simulink model "PRACTICA_03_P1_00"  (R2022a)
settings: Solver=VariableStepAuto  StartTime=0.0  StopTime=10.0  RelTol=1e-3
undefined symbols (not defined in the file or in its folder): xc7z010iclg225
libraries: hdlBasic x889, vmcUtilities x1
(part 2 of 4)

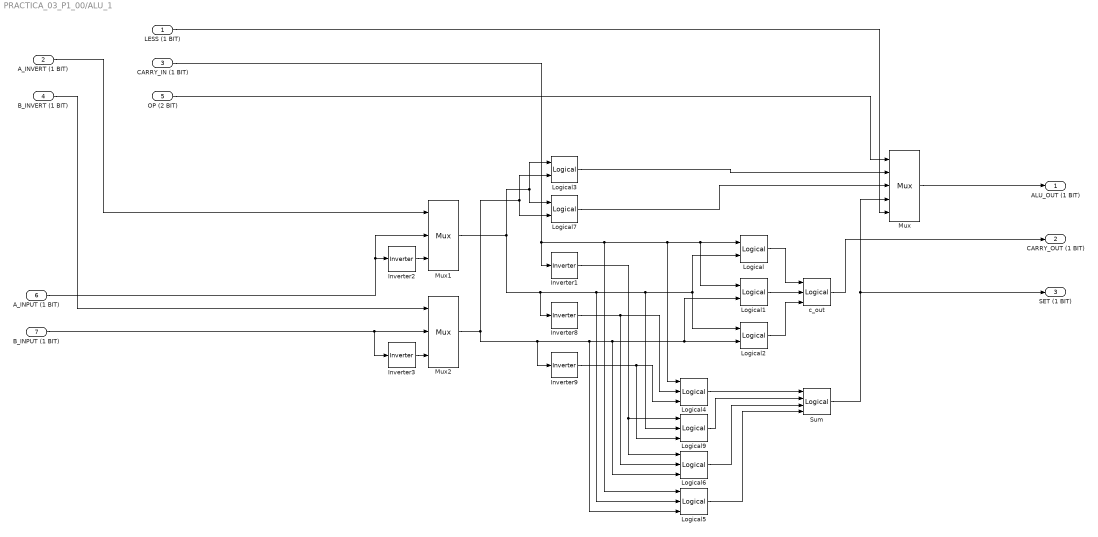
== system PRACTICA_03_P1_00/ALU_1 ==
  LESS (1 BIT) : Inport
  A_INVERT (1 BIT) : Inport  Port=2
  CARRY_IN (1 BIT) : Inport  Port=3
  B_INVERT (1 BIT) : Inport  Port=4
  OP (2 BIT) : Inport  Port=5
  A_INPUT (1 BIT) : Inport  Port=6
  B_INPUT (1 BIT) : Inport  Port=7
  Inverter{1..3,8..9} (5 alike) : hdlBasic/Inverter  en=off  latency=0  XmcBlockStatus=1  maskContainerNames=group2  block_type=inv  block_config=sysgen:Inverter_config
  Logical{,1..3} (4 alike) : hdlBasic/Logical  logical_function=AND  inputs=2  en=off  latency=0  precision=Full  arith_type=Unsigned  n_bits=16  bin_pt=0  align_bp=on  overflow=[]  quantization=[]  XmcBlockStatus=1  maskContainerNames=tabcontainer1  block_type=logical  block_config=sysgen:Logical_config
  Logical{4..6,9} (4 alike) : hdlBasic/Logical  logical_function=AND  inputs=3  en=off  latency=0  precision=Full  arith_type=Unsigned  n_bits=16  bin_pt=0  align_bp=on  overflow=[]  quantization=[]  XmcBlockStatus=1  maskContainerNames=tabcontainer1  block_type=logical  block_config=sysgen:Logical_config
  Logical7 : hdlBasic/Logical  logical_function=OR  inputs=2  en=off  latency=0  precision=Full  arith_type=Unsigned  n_bits=16  bin_pt=0  align_bp=on  overflow=[]  quantization=[]  XmcBlockStatus=1  maskContainerNames=tabcontainer1  block_type=logical  block_config=sysgen:Logical_config
  Mux : hdlBasic/Mux  inputs=4  en=off  latency=0  precision=Full  arith_type=Unsigned  n_bits=16  bin_pt=14  quantization=Truncate  overflow=Wrap  XmcBlockStatus=1  maskContainerNames=tabcontainer1  block_type=mux  block_config=sysgen:Mux_config
  Mux1 : hdlBasic/Mux  inputs=2  en=off  latency=0  precision=Full  arith_type=Unsigned  n_bits=16  bin_pt=14  quantization=Truncate  overflow=Wrap  XmcBlockStatus=1  maskContainerNames=tabcontainer1  block_type=mux  block_config=sysgen:Mux_config
  Mux2 : hdlBasic/Mux  inputs=2  en=off  latency=0  precision=Full  arith_type=Unsigned  n_bits=16  bin_pt=14  quantization=Truncate  overflow=Wrap  XmcBlockStatus=1  maskContainerNames=tabcontainer1  block_type=mux  block_config=sysgen:Mux_config
  Sum : hdlBasic/Logical  logical_function=OR  inputs=4  en=off  latency=0  precision=Full  arith_type=Unsigned  n_bits=16  bin_pt=0  align_bp=on  overflow=[]  quantization=[]  XmcBlockStatus=1  maskContainerNames=tabcontainer1  block_type=logical  block_config=sysgen:Logical_config
  c_out : hdlBasic/Logical  logical_function=OR  inputs=3  en=off  latency=0  precision=Full  arith_type=Unsigned  n_bits=16  bin_pt=0  align_bp=on  overflow=[]  quantization=[]  XmcBlockStatus=1  maskContainerNames=tabcontainer1  block_type=logical  block_config=sysgen:Logical_config
  ALU_OUT (1 BIT) : Outport
  CARRY_OUT (1 BIT) : Outport  Port=2
  SET (1 BIT) : Outport  Port=3
  wires:
  Mux1/1 -> Logical3/1, Logical7/1, Inverter8/1, Logical5/2, Logical/2, Logical2/1, Logical9/2
  Logical1/1 -> c_out/2
  Inverter8/1 -> Logical6/2, Logical4/2
  A_INPUT (1 BIT)/1 -> Mux1/2, Inverter2/1
  CARRY_IN (1 BIT)/1 -> Inverter1/1, Logical5/1, Logical4/1, Logical1/1, Logical/1
  Mux2/1 -> Logical5/3, Logical6/3, Logical1/2, Logical2/2, Inverter9/1, Logical3/2, Logical7/2
  Inverter2/1 -> Mux1/3
  Inverter1/1 -> Logical6/1, Logical9/1
  Logical6/1 -> Sum/3
  B_INPUT (1 BIT)/1 -> Inverter3/1, Mux2/2
  Logical9/1 -> Sum/2
  Sum/1 -> SET (1 BIT)/1, Mux/4
  Logical4/1 -> Sum/1
  Inverter3/1 -> Mux2/3
  Logical7/1 -> Mux/3
  Logical/1 -> c_out/1
  Logical5/1 -> Sum/4
  Logical3/1 -> Mux/2
  Inverter9/1 -> Logical9/3, Logical4/3
  Mux/1 -> ALU_OUT (1 BIT)/1
  Logical2/1 -> c_out/3
  OP (2 BIT)/1 -> Mux/1
  A_INVERT (1 BIT)/1 -> Mux1/1
  B_INVERT (1 BIT)/1 -> Mux2/1
  c_out/1 -> CARRY_OUT (1 BIT)/1
  LESS (1 BIT)/1 -> Mux/5

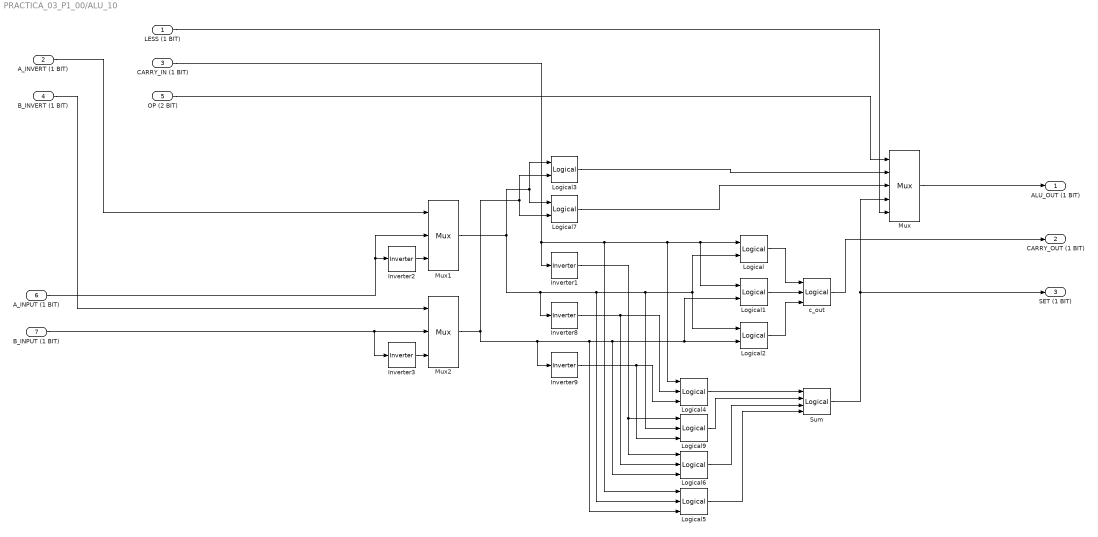
== system PRACTICA_03_P1_00/ALU_10 ==
  LESS (1 BIT) : Inport
  A_INVERT (1 BIT) : Inport  Port=2
  CARRY_IN (1 BIT) : Inport  Port=3
  B_INVERT (1 BIT) : Inport  Port=4
  OP (2 BIT) : Inport  Port=5
  A_INPUT (1 BIT) : Inport  Port=6
  B_INPUT (1 BIT) : Inport  Port=7
  Inverter{1..3,8..9} (5 alike) : hdlBasic/Inverter  en=off  latency=0  XmcBlockStatus=1  maskContainerNames=group2  block_type=inv  block_config=sysgen:Inverter_config
  Logical{,1..3} (4 alike) : hdlBasic/Logical  logical_function=AND  inputs=2  en=off  latency=0  precision=Full  arith_type=Unsigned  n_bits=16  bin_pt=0  align_bp=on  overflow=[]  quantization=[]  XmcBlockStatus=1  maskContainerNames=tabcontainer1  block_type=logical  block_config=sysgen:Logical_config
  Logical{4..6,9} (4 alike) : hdlBasic/Logical  logical_function=AND  inputs=3  en=off  latency=0  precision=Full  arith_type=Unsigned  n_bits=16  bin_pt=0  align_bp=on  overflow=[]  quantization=[]  XmcBlockStatus=1  maskContainerNames=tabcontainer1  block_type=logical  block_config=sysgen:Logical_config
  Logical7 : hdlBasic/Logical  logical_function=OR  inputs=2  en=off  latency=0  precision=Full  arith_type=Unsigned  n_bits=16  bin_pt=0  align_bp=on  overflow=[]  quantization=[]  XmcBlockStatus=1  maskContainerNames=tabcontainer1  block_type=logical  block_config=sysgen:Logical_config
  Mux : hdlBasic/Mux  inputs=4  en=off  latency=0  precision=Full  arith_type=Unsigned  n_bits=16  bin_pt=14  quantization=Truncate  overflow=Wrap  XmcBlockStatus=1  maskContainerNames=tabcontainer1  block_type=mux  block_config=sysgen:Mux_config
  Mux1 : hdlBasic/Mux  inputs=2  en=off  latency=0  precision=Full  arith_type=Unsigned  n_bits=16  bin_pt=14  quantization=Truncate  overflow=Wrap  XmcBlockStatus=1  maskContainerNames=tabcontainer1  block_type=mux  block_config=sysgen:Mux_config
  Mux2 : hdlBasic/Mux  inputs=2  en=off  latency=0  precision=Full  arith_type=Unsigned  n_bits=16  bin_pt=14  quantization=Truncate  overflow=Wrap  XmcBlockStatus=1  maskContainerNames=tabcontainer1  block_type=mux  block_config=sysgen:Mux_config
  Sum : hdlBasic/Logical  logical_function=OR  inputs=4  en=off  latency=0  precision=Full  arith_type=Unsigned  n_bits=16  bin_pt=0  align_bp=on  overflow=[]  quantization=[]  XmcBlockStatus=1  maskContainerNames=tabcontainer1  block_type=logical  block_config=sysgen:Logical_config
  c_out : hdlBasic/Logical  logical_function=OR  inputs=3  en=off  latency=0  precision=Full  arith_type=Unsigned  n_bits=16  bin_pt=0  align_bp=on  overflow=[]  quantization=[]  XmcBlockStatus=1  maskContainerNames=tabcontainer1  block_type=logical  block_config=sysgen:Logical_config
  ALU_OUT (1 BIT) : Outport
  CARRY_OUT (1 BIT) : Outport  Port=2
  SET (1 BIT) : Outport  Port=3
  wires:
  Mux1/1 -> Logical3/1, Logical7/1, Inverter8/1, Logical5/2, Logical/2, Logical2/1, Logical9/2
  Logical1/1 -> c_out/2
  Inverter8/1 -> Logical6/2, Logical4/2
  A_INPUT (1 BIT)/1 -> Mux1/2, Inverter2/1
  CARRY_IN (1 BIT)/1 -> Inverter1/1, Logical5/1, Logical4/1, Logical1/1, Logical/1
  Mux2/1 -> Logical5/3, Logical6/3, Logical1/2, Logical2/2, Inverter9/1, Logical3/2, Logical7/2
  Inverter2/1 -> Mux1/3
  Inverter1/1 -> Logical6/1, Logical9/1
  Logical6/1 -> Sum/3
  B_INPUT (1 BIT)/1 -> Inverter3/1, Mux2/2
  Logical9/1 -> Sum/2
  Sum/1 -> SET (1 BIT)/1, Mux/4
  Logical4/1 -> Sum/1
  Inverter3/1 -> Mux2/3
  Logical7/1 -> Mux/3
  Logical/1 -> c_out/1
  Logical5/1 -> Sum/4
  Logical3/1 -> Mux/2
  Inverter9/1 -> Logical9/3, Logical4/3
  Mux/1 -> ALU_OUT (1 BIT)/1
  Logical2/1 -> c_out/3
  OP (2 BIT)/1 -> Mux/1
  A_INVERT (1 BIT)/1 -> Mux1/1
  B_INVERT (1 BIT)/1 -> Mux2/1
  c_out/1 -> CARRY_OUT (1 BIT)/1
  LESS (1 BIT)/1 -> Mux/5

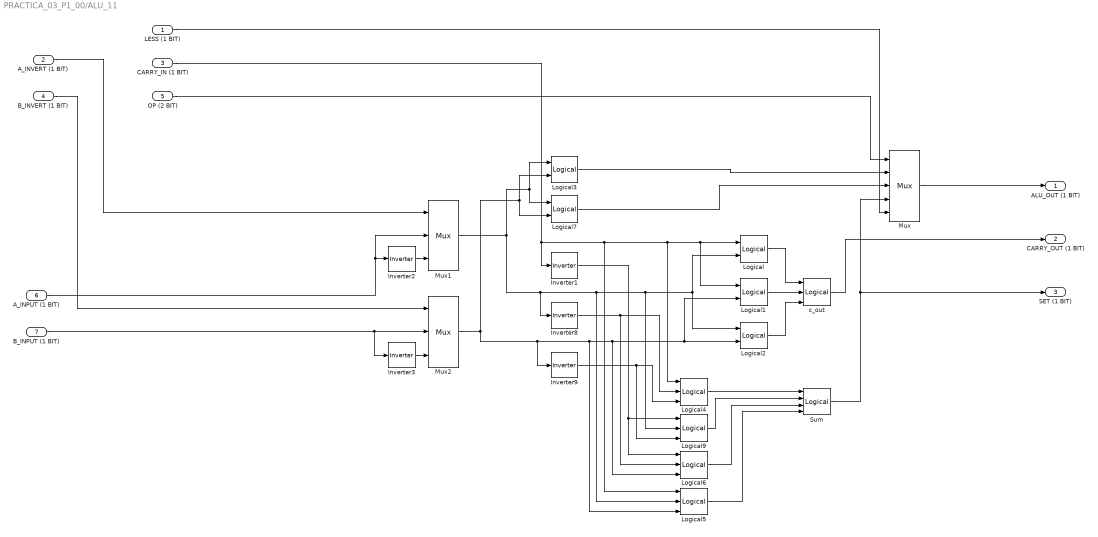
== system PRACTICA_03_P1_00/ALU_11 ==
  LESS (1 BIT) : Inport
  A_INVERT (1 BIT) : Inport  Port=2
  CARRY_IN (1 BIT) : Inport  Port=3
  B_INVERT (1 BIT) : Inport  Port=4
  OP (2 BIT) : Inport  Port=5
  A_INPUT (1 BIT) : Inport  Port=6
  B_INPUT (1 BIT) : Inport  Port=7
  Inverter{1..3,8..9} (5 alike) : hdlBasic/Inverter  en=off  latency=0  XmcBlockStatus=1  maskContainerNames=group2  block_type=inv  block_config=sysgen:Inverter_config
  Logical{,1..3} (4 alike) : hdlBasic/Logical  logical_function=AND  inputs=2  en=off  latency=0  precision=Full  arith_type=Unsigned  n_bits=16  bin_pt=0  align_bp=on  overflow=[]  quantization=[]  XmcBlockStatus=1  maskContainerNames=tabcontainer1  block_type=logical  block_config=sysgen:Logical_config
  Logical{4..6,9} (4 alike) : hdlBasic/Logical  logical_function=AND  inputs=3  en=off  latency=0  precision=Full  arith_type=Unsigned  n_bits=16  bin_pt=0  align_bp=on  overflow=[]  quantization=[]  XmcBlockStatus=1  maskContainerNames=tabcontainer1  block_type=logical  block_config=sysgen:Logical_config
  Logical7 : hdlBasic/Logical  logical_function=OR  inputs=2  en=off  latency=0  precision=Full  arith_type=Unsigned  n_bits=16  bin_pt=0  align_bp=on  overflow=[]  quantization=[]  XmcBlockStatus=1  maskContainerNames=tabcontainer1  block_type=logical  block_config=sysgen:Logical_config
  Mux : hdlBasic/Mux  inputs=4  en=off  latency=0  precision=Full  arith_type=Unsigned  n_bits=16  bin_pt=14  quantization=Truncate  overflow=Wrap  XmcBlockStatus=1  maskContainerNames=tabcontainer1  block_type=mux  block_config=sysgen:Mux_config
  Mux1 : hdlBasic/Mux  inputs=2  en=off  latency=0  precision=Full  arith_type=Unsigned  n_bits=16  bin_pt=14  quantization=Truncate  overflow=Wrap  XmcBlockStatus=1  maskContainerNames=tabcontainer1  block_type=mux  block_config=sysgen:Mux_config
  Mux2 : hdlBasic/Mux  inputs=2  en=off  latency=0  precision=Full  arith_type=Unsigned  n_bits=16  bin_pt=14  quantization=Truncate  overflow=Wrap  XmcBlockStatus=1  maskContainerNames=tabcontainer1  block_type=mux  block_config=sysgen:Mux_config
  Sum : hdlBasic/Logical  logical_function=OR  inputs=4  en=off  latency=0  precision=Full  arith_type=Unsigned  n_bits=16  bin_pt=0  align_bp=on  overflow=[]  quantization=[]  XmcBlockStatus=1  maskContainerNames=tabcontainer1  block_type=logical  block_config=sysgen:Logical_config
  c_out : hdlBasic/Logical  logical_function=OR  inputs=3  en=off  latency=0  precision=Full  arith_type=Unsigned  n_bits=16  bin_pt=0  align_bp=on  overflow=[]  quantization=[]  XmcBlockStatus=1  maskContainerNames=tabcontainer1  block_type=logical  block_config=sysgen:Logical_config
  ALU_OUT (1 BIT) : Outport
  CARRY_OUT (1 BIT) : Outport  Port=2
  SET (1 BIT) : Outport  Port=3
  wires:
  Mux1/1 -> Logical3/1, Logical7/1, Inverter8/1, Logical5/2, Logical/2, Logical2/1, Logical9/2
  Logical1/1 -> c_out/2
  Inverter8/1 -> Logical6/2, Logical4/2
  A_INPUT (1 BIT)/1 -> Mux1/2, Inverter2/1
  CARRY_IN (1 BIT)/1 -> Inverter1/1, Logical5/1, Logical4/1, Logical1/1, Logical/1
  Mux2/1 -> Logical5/3, Logical6/3, Logical1/2, Logical2/2, Inverter9/1, Logical3/2, Logical7/2
  Inverter2/1 -> Mux1/3
  Inverter1/1 -> Logical6/1, Logical9/1
  Logical6/1 -> Sum/3
  B_INPUT (1 BIT)/1 -> Inverter3/1, Mux2/2
  Logical9/1 -> Sum/2
  Sum/1 -> SET (1 BIT)/1, Mux/4
  Logical4/1 -> Sum/1
  Inverter3/1 -> Mux2/3
  Logical7/1 -> Mux/3
  Logical/1 -> c_out/1
  Logical5/1 -> Sum/4
  Logical3/1 -> Mux/2
  Inverter9/1 -> Logical9/3, Logical4/3
  Mux/1 -> ALU_OUT (1 BIT)/1
  Logical2/1 -> c_out/3
  OP (2 BIT)/1 -> Mux/1
  A_INVERT (1 BIT)/1 -> Mux1/1
  B_INVERT (1 BIT)/1 -> Mux2/1
  c_out/1 -> CARRY_OUT (1 BIT)/1
  LESS (1 BIT)/1 -> Mux/5

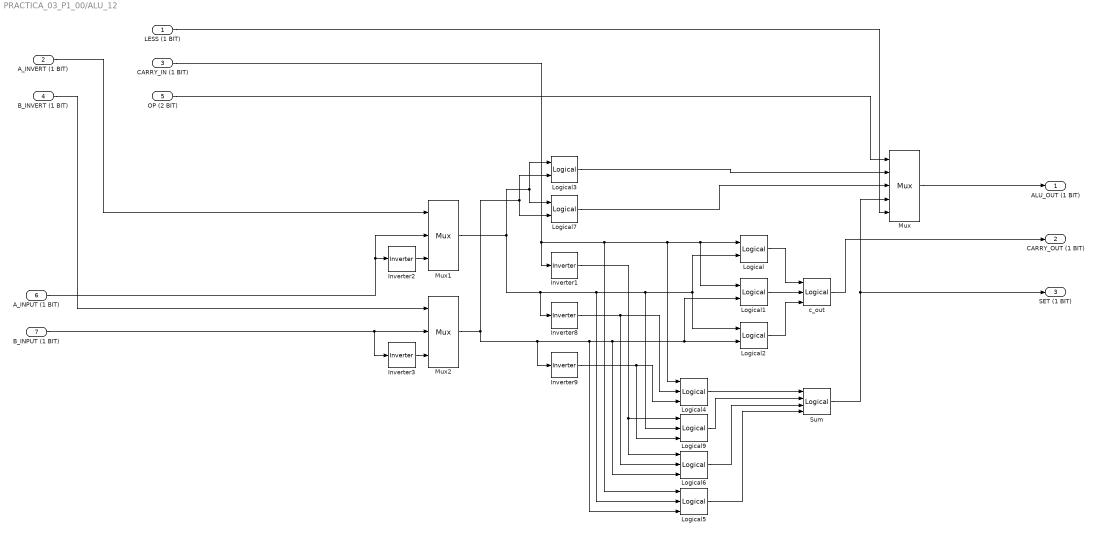
== system PRACTICA_03_P1_00/ALU_12 ==
  LESS (1 BIT) : Inport
  A_INVERT (1 BIT) : Inport  Port=2
  CARRY_IN (1 BIT) : Inport  Port=3
  B_INVERT (1 BIT) : Inport  Port=4
  OP (2 BIT) : Inport  Port=5
  A_INPUT (1 BIT) : Inport  Port=6
  B_INPUT (1 BIT) : Inport  Port=7
  Inverter{1..3,8..9} (5 alike) : hdlBasic/Inverter  en=off  latency=0  XmcBlockStatus=1  maskContainerNames=group2  block_type=inv  block_config=sysgen:Inverter_config
  Logical{,1..3} (4 alike) : hdlBasic/Logical  logical_function=AND  inputs=2  en=off  latency=0  precision=Full  arith_type=Unsigned  n_bits=16  bin_pt=0  align_bp=on  overflow=[]  quantization=[]  XmcBlockStatus=1  maskContainerNames=tabcontainer1  block_type=logical  block_config=sysgen:Logical_config
  Logical{4..6,9} (4 alike) : hdlBasic/Logical  logical_function=AND  inputs=3  en=off  latency=0  precision=Full  arith_type=Unsigned  n_bits=16  bin_pt=0  align_bp=on  overflow=[]  quantization=[]  XmcBlockStatus=1  maskContainerNames=tabcontainer1  block_type=logical  block_config=sysgen:Logical_config
  Logical7 : hdlBasic/Logical  logical_function=OR  inputs=2  en=off  latency=0  precision=Full  arith_type=Unsigned  n_bits=16  bin_pt=0  align_bp=on  overflow=[]  quantization=[]  XmcBlockStatus=1  maskContainerNames=tabcontainer1  block_type=logical  block_config=sysgen:Logical_config
  Mux : hdlBasic/Mux  inputs=4  en=off  latency=0  precision=Full  arith_type=Unsigned  n_bits=16  bin_pt=14  quantization=Truncate  overflow=Wrap  XmcBlockStatus=1  maskContainerNames=tabcontainer1  block_type=mux  block_config=sysgen:Mux_config
  Mux1 : hdlBasic/Mux  inputs=2  en=off  latency=0  precision=Full  arith_type=Unsigned  n_bits=16  bin_pt=14  quantization=Truncate  overflow=Wrap  XmcBlockStatus=1  maskContainerNames=tabcontainer1  block_type=mux  block_config=sysgen:Mux_config
  Mux2 : hdlBasic/Mux  inputs=2  en=off  latency=0  precision=Full  arith_type=Unsigned  n_bits=16  bin_pt=14  quantization=Truncate  overflow=Wrap  XmcBlockStatus=1  maskContainerNames=tabcontainer1  block_type=mux  block_config=sysgen:Mux_config
  Sum : hdlBasic/Logical  logical_function=OR  inputs=4  en=off  latency=0  precision=Full  arith_type=Unsigned  n_bits=16  bin_pt=0  align_bp=on  overflow=[]  quantization=[]  XmcBlockStatus=1  maskContainerNames=tabcontainer1  block_type=logical  block_config=sysgen:Logical_config
  c_out : hdlBasic/Logical  logical_function=OR  inputs=3  en=off  latency=0  precision=Full  arith_type=Unsigned  n_bits=16  bin_pt=0  align_bp=on  overflow=[]  quantization=[]  XmcBlockStatus=1  maskContainerNames=tabcontainer1  block_type=logical  block_config=sysgen:Logical_config
  ALU_OUT (1 BIT) : Outport
  CARRY_OUT (1 BIT) : Outport  Port=2
  SET (1 BIT) : Outport  Port=3
  wires:
  Mux1/1 -> Logical3/1, Logical7/1, Inverter8/1, Logical5/2, Logical/2, Logical2/1, Logical9/2
  Logical1/1 -> c_out/2
  Inverter8/1 -> Logical6/2, Logical4/2
  A_INPUT (1 BIT)/1 -> Mux1/2, Inverter2/1
  CARRY_IN (1 BIT)/1 -> Inverter1/1, Logical5/1, Logical4/1, Logical1/1, Logical/1
  Mux2/1 -> Logical5/3, Logical6/3, Logical1/2, Logical2/2, Inverter9/1, Logical3/2, Logical7/2
  Inverter2/1 -> Mux1/3
  Inverter1/1 -> Logical6/1, Logical9/1
  Logical6/1 -> Sum/3
  B_INPUT (1 BIT)/1 -> Inverter3/1, Mux2/2
  Logical9/1 -> Sum/2
  Sum/1 -> SET (1 BIT)/1, Mux/4
  Logical4/1 -> Sum/1
  Inverter3/1 -> Mux2/3
  Logical7/1 -> Mux/3
  Logical/1 -> c_out/1
  Logical5/1 -> Sum/4
  Logical3/1 -> Mux/2
  Inverter9/1 -> Logical9/3, Logical4/3
  Mux/1 -> ALU_OUT (1 BIT)/1
  Logical2/1 -> c_out/3
  OP (2 BIT)/1 -> Mux/1
  A_INVERT (1 BIT)/1 -> Mux1/1
  B_INVERT (1 BIT)/1 -> Mux2/1
  c_out/1 -> CARRY_OUT (1 BIT)/1
  LESS (1 BIT)/1 -> Mux/5

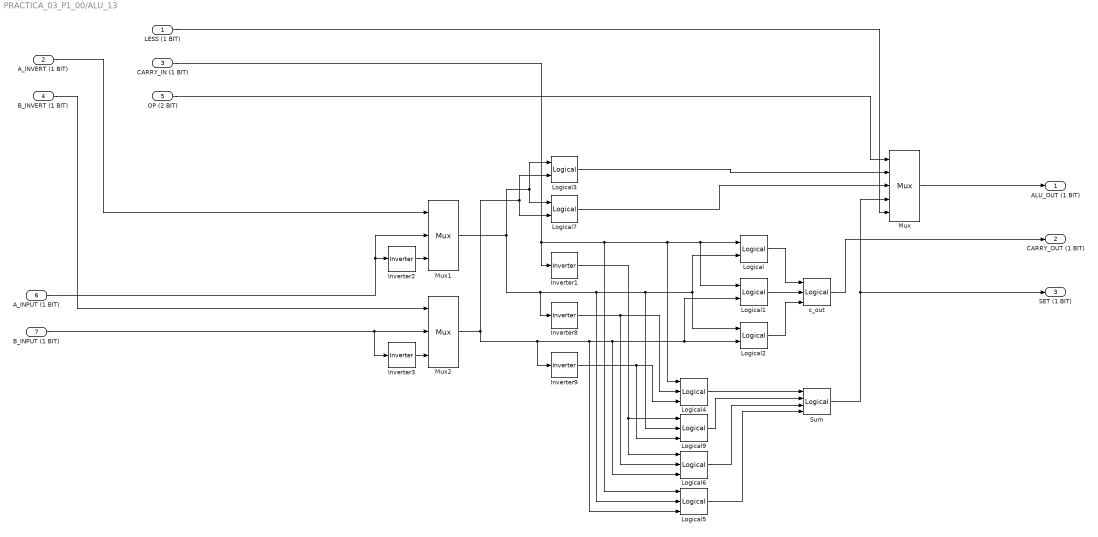
== system PRACTICA_03_P1_00/ALU_13 ==
  LESS (1 BIT) : Inport
  A_INVERT (1 BIT) : Inport  Port=2
  CARRY_IN (1 BIT) : Inport  Port=3
  B_INVERT (1 BIT) : Inport  Port=4
  OP (2 BIT) : Inport  Port=5
  A_INPUT (1 BIT) : Inport  Port=6
  B_INPUT (1 BIT) : Inport  Port=7
  Inverter{1..3,8..9} (5 alike) : hdlBasic/Inverter  en=off  latency=0  XmcBlockStatus=1  maskContainerNames=group2  block_type=inv  block_config=sysgen:Inverter_config
  Logical{,1..3} (4 alike) : hdlBasic/Logical  logical_function=AND  inputs=2  en=off  latency=0  precision=Full  arith_type=Unsigned  n_bits=16  bin_pt=0  align_bp=on  overflow=[]  quantization=[]  XmcBlockStatus=1  maskContainerNames=tabcontainer1  block_type=logical  block_config=sysgen:Logical_config
  Logical{4..6,9} (4 alike) : hdlBasic/Logical  logical_function=AND  inputs=3  en=off  latency=0  precision=Full  arith_type=Unsigned  n_bits=16  bin_pt=0  align_bp=on  overflow=[]  quantization=[]  XmcBlockStatus=1  maskContainerNames=tabcontainer1  block_type=logical  block_config=sysgen:Logical_config
  Logical7 : hdlBasic/Logical  logical_function=OR  inputs=2  en=off  latency=0  precision=Full  arith_type=Unsigned  n_bits=16  bin_pt=0  align_bp=on  overflow=[]  quantization=[]  XmcBlockStatus=1  maskContainerNames=tabcontainer1  block_type=logical  block_config=sysgen:Logical_config
  Mux : hdlBasic/Mux  inputs=4  en=off  latency=0  precision=Full  arith_type=Unsigned  n_bits=16  bin_pt=14  quantization=Truncate  overflow=Wrap  XmcBlockStatus=1  maskContainerNames=tabcontainer1  block_type=mux  block_config=sysgen:Mux_config
  Mux1 : hdlBasic/Mux  inputs=2  en=off  latency=0  precision=Full  arith_type=Unsigned  n_bits=16  bin_pt=14  quantization=Truncate  overflow=Wrap  XmcBlockStatus=1  maskContainerNames=tabcontainer1  block_type=mux  block_config=sysgen:Mux_config
  Mux2 : hdlBasic/Mux  inputs=2  en=off  latency=0  precision=Full  arith_type=Unsigned  n_bits=16  bin_pt=14  quantization=Truncate  overflow=Wrap  XmcBlockStatus=1  maskContainerNames=tabcontainer1  block_type=mux  block_config=sysgen:Mux_config
  Sum : hdlBasic/Logical  logical_function=OR  inputs=4  en=off  latency=0  precision=Full  arith_type=Unsigned  n_bits=16  bin_pt=0  align_bp=on  overflow=[]  quantization=[]  XmcBlockStatus=1  maskContainerNames=tabcontainer1  block_type=logical  block_config=sysgen:Logical_config
  c_out : hdlBasic/Logical  logical_function=OR  inputs=3  en=off  latency=0  precision=Full  arith_type=Unsigned  n_bits=16  bin_pt=0  align_bp=on  overflow=[]  quantization=[]  XmcBlockStatus=1  maskContainerNames=tabcontainer1  block_type=logical  block_config=sysgen:Logical_config
  ALU_OUT (1 BIT) : Outport
  CARRY_OUT (1 BIT) : Outport  Port=2
  SET (1 BIT) : Outport  Port=3
  wires:
  Mux1/1 -> Logical3/1, Logical7/1, Inverter8/1, Logical5/2, Logical/2, Logical2/1, Logical9/2
  Logical1/1 -> c_out/2
  Inverter8/1 -> Logical6/2, Logical4/2
  A_INPUT (1 BIT)/1 -> Mux1/2, Inverter2/1
  CARRY_IN (1 BIT)/1 -> Inverter1/1, Logical5/1, Logical4/1, Logical1/1, Logical/1
  Mux2/1 -> Logical5/3, Logical6/3, Logical1/2, Logical2/2, Inverter9/1, Logical3/2, Logical7/2
  Inverter2/1 -> Mux1/3
  Inverter1/1 -> Logical6/1, Logical9/1
  Logical6/1 -> Sum/3
  B_INPUT (1 BIT)/1 -> Inverter3/1, Mux2/2
  Logical9/1 -> Sum/2
  Sum/1 -> SET (1 BIT)/1, Mux/4
  Logical4/1 -> Sum/1
  Inverter3/1 -> Mux2/3
  Logical7/1 -> Mux/3
  Logical/1 -> c_out/1
  Logical5/1 -> Sum/4
  Logical3/1 -> Mux/2
  Inverter9/1 -> Logical9/3, Logical4/3
  Mux/1 -> ALU_OUT (1 BIT)/1
  Logical2/1 -> c_out/3
  OP (2 BIT)/1 -> Mux/1
  A_INVERT (1 BIT)/1 -> Mux1/1
  B_INVERT (1 BIT)/1 -> Mux2/1
  c_out/1 -> CARRY_OUT (1 BIT)/1
  LESS (1 BIT)/1 -> Mux/5

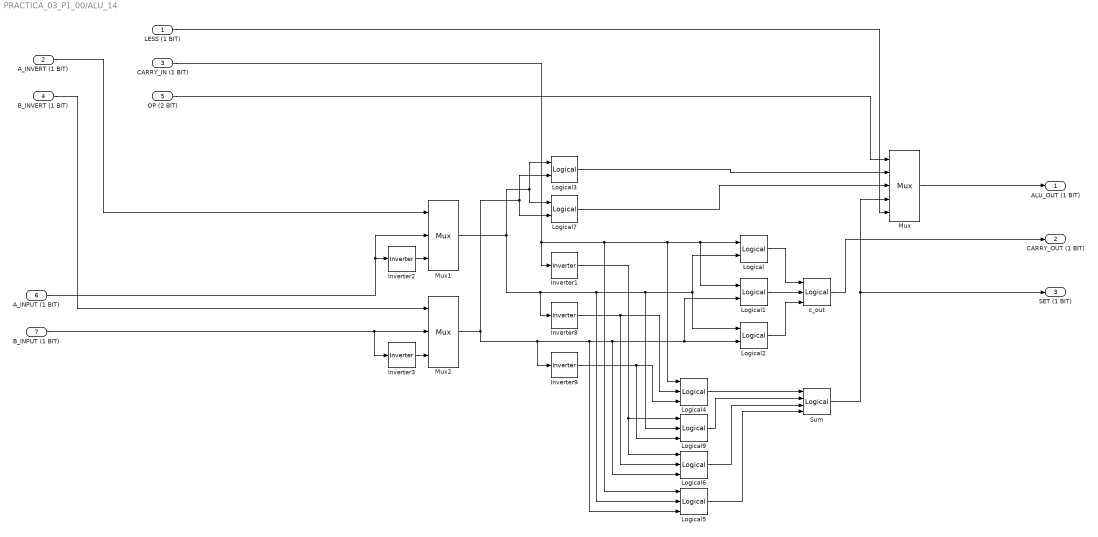
== system PRACTICA_03_P1_00/ALU_14 ==
  LESS (1 BIT) : Inport
  A_INVERT (1 BIT) : Inport  Port=2
  CARRY_IN (1 BIT) : Inport  Port=3
  B_INVERT (1 BIT) : Inport  Port=4
  OP (2 BIT) : Inport  Port=5
  A_INPUT (1 BIT) : Inport  Port=6
  B_INPUT (1 BIT) : Inport  Port=7
  Inverter{1..3,8..9} (5 alike) : hdlBasic/Inverter  en=off  latency=0  XmcBlockStatus=1  maskContainerNames=group2  block_type=inv  block_config=sysgen:Inverter_config
  Logical{,1..3} (4 alike) : hdlBasic/Logical  logical_function=AND  inputs=2  en=off  latency=0  precision=Full  arith_type=Unsigned  n_bits=16  bin_pt=0  align_bp=on  overflow=[]  quantization=[]  XmcBlockStatus=1  maskContainerNames=tabcontainer1  block_type=logical  block_config=sysgen:Logical_config
  Logical{4..6,9} (4 alike) : hdlBasic/Logical  logical_function=AND  inputs=3  en=off  latency=0  precision=Full  arith_type=Unsigned  n_bits=16  bin_pt=0  align_bp=on  overflow=[]  quantization=[]  XmcBlockStatus=1  maskContainerNames=tabcontainer1  block_type=logical  block_config=sysgen:Logical_config
  Logical7 : hdlBasic/Logical  logical_function=OR  inputs=2  en=off  latency=0  precision=Full  arith_type=Unsigned  n_bits=16  bin_pt=0  align_bp=on  overflow=[]  quantization=[]  XmcBlockStatus=1  maskContainerNames=tabcontainer1  block_type=logical  block_config=sysgen:Logical_config
  Mux : hdlBasic/Mux  inputs=4  en=off  latency=0  precision=Full  arith_type=Unsigned  n_bits=16  bin_pt=14  quantization=Truncate  overflow=Wrap  XmcBlockStatus=1  maskContainerNames=tabcontainer1  block_type=mux  block_config=sysgen:Mux_config
  Mux1 : hdlBasic/Mux  inputs=2  en=off  latency=0  precision=Full  arith_type=Unsigned  n_bits=16  bin_pt=14  quantization=Truncate  overflow=Wrap  XmcBlockStatus=1  maskContainerNames=tabcontainer1  block_type=mux  block_config=sysgen:Mux_config
  Mux2 : hdlBasic/Mux  inputs=2  en=off  latency=0  precision=Full  arith_type=Unsigned  n_bits=16  bin_pt=14  quantization=Truncate  overflow=Wrap  XmcBlockStatus=1  maskContainerNames=tabcontainer1  block_type=mux  block_config=sysgen:Mux_config
  Sum : hdlBasic/Logical  logical_function=OR  inputs=4  en=off  latency=0  precision=Full  arith_type=Unsigned  n_bits=16  bin_pt=0  align_bp=on  overflow=[]  quantization=[]  XmcBlockStatus=1  maskContainerNames=tabcontainer1  block_type=logical  block_config=sysgen:Logical_config
  c_out : hdlBasic/Logical  logical_function=OR  inputs=3  en=off  latency=0  precision=Full  arith_type=Unsigned  n_bits=16  bin_pt=0  align_bp=on  overflow=[]  quantization=[]  XmcBlockStatus=1  maskContainerNames=tabcontainer1  block_type=logical  block_config=sysgen:Logical_config
  ALU_OUT (1 BIT) : Outport
  CARRY_OUT (1 BIT) : Outport  Port=2
  SET (1 BIT) : Outport  Port=3
  wires:
  Mux1/1 -> Logical3/1, Logical7/1, Inverter8/1, Logical5/2, Logical/2, Logical2/1, Logical9/2
  Logical1/1 -> c_out/2
  Inverter8/1 -> Logical6/2, Logical4/2
  A_INPUT (1 BIT)/1 -> Mux1/2, Inverter2/1
  CARRY_IN (1 BIT)/1 -> Inverter1/1, Logical5/1, Logical4/1, Logical1/1, Logical/1
  Mux2/1 -> Logical5/3, Logical6/3, Logical1/2, Logical2/2, Inverter9/1, Logical3/2, Logical7/2
  Inverter2/1 -> Mux1/3
  Inverter1/1 -> Logical6/1, Logical9/1
  Logical6/1 -> Sum/3
  B_INPUT (1 BIT)/1 -> Inverter3/1, Mux2/2
  Logical9/1 -> Sum/2
  Sum/1 -> SET (1 BIT)/1, Mux/4
  Logical4/1 -> Sum/1
  Inverter3/1 -> Mux2/3
  Logical7/1 -> Mux/3
  Logical/1 -> c_out/1
  Logical5/1 -> Sum/4
  Logical3/1 -> Mux/2
  Inverter9/1 -> Logical9/3, Logical4/3
  Mux/1 -> ALU_OUT (1 BIT)/1
  Logical2/1 -> c_out/3
  OP (2 BIT)/1 -> Mux/1
  A_INVERT (1 BIT)/1 -> Mux1/1
  B_INVERT (1 BIT)/1 -> Mux2/1
  c_out/1 -> CARRY_OUT (1 BIT)/1
  LESS (1 BIT)/1 -> Mux/5

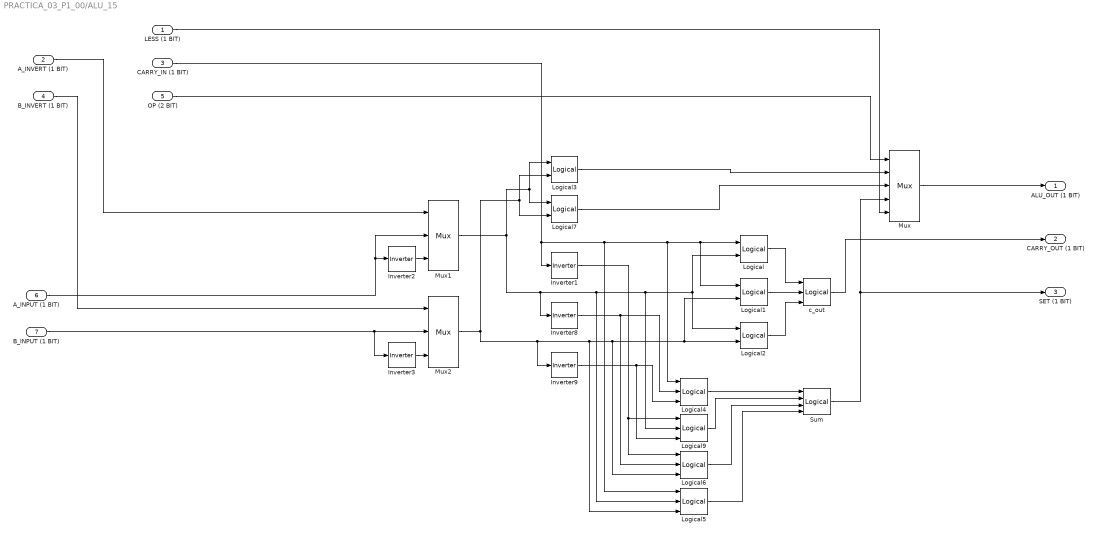
== system PRACTICA_03_P1_00/ALU_15 ==
  LESS (1 BIT) : Inport
  A_INVERT (1 BIT) : Inport  Port=2
  CARRY_IN (1 BIT) : Inport  Port=3
  B_INVERT (1 BIT) : Inport  Port=4
  OP (2 BIT) : Inport  Port=5
  A_INPUT (1 BIT) : Inport  Port=6
  B_INPUT (1 BIT) : Inport  Port=7
  Inverter{1..3,8..9} (5 alike) : hdlBasic/Inverter  en=off  latency=0  XmcBlockStatus=1  maskContainerNames=group2  block_type=inv  block_config=sysgen:Inverter_config
  Logical{,1..3} (4 alike) : hdlBasic/Logical  logical_function=AND  inputs=2  en=off  latency=0  precision=Full  arith_type=Unsigned  n_bits=16  bin_pt=0  align_bp=on  overflow=[]  quantization=[]  XmcBlockStatus=1  maskContainerNames=tabcontainer1  block_type=logical  block_config=sysgen:Logical_config
  Logical{4..6,9} (4 alike) : hdlBasic/Logical  logical_function=AND  inputs=3  en=off  latency=0  precision=Full  arith_type=Unsigned  n_bits=16  bin_pt=0  align_bp=on  overflow=[]  quantization=[]  XmcBlockStatus=1  maskContainerNames=tabcontainer1  block_type=logical  block_config=sysgen:Logical_config
  Logical7 : hdlBasic/Logical  logical_function=OR  inputs=2  en=off  latency=0  precision=Full  arith_type=Unsigned  n_bits=16  bin_pt=0  align_bp=on  overflow=[]  quantization=[]  XmcBlockStatus=1  maskContainerNames=tabcontainer1  block_type=logical  block_config=sysgen:Logical_config
  Mux : hdlBasic/Mux  inputs=4  en=off  latency=0  precision=Full  arith_type=Unsigned  n_bits=16  bin_pt=14  quantization=Truncate  overflow=Wrap  XmcBlockStatus=1  maskContainerNames=tabcontainer1  block_type=mux  block_config=sysgen:Mux_config
  Mux1 : hdlBasic/Mux  inputs=2  en=off  latency=0  precision=Full  arith_type=Unsigned  n_bits=16  bin_pt=14  quantization=Truncate  overflow=Wrap  XmcBlockStatus=1  maskContainerNames=tabcontainer1  block_type=mux  block_config=sysgen:Mux_config
  Mux2 : hdlBasic/Mux  inputs=2  en=off  latency=0  precision=Full  arith_type=Unsigned  n_bits=16  bin_pt=14  quantization=Truncate  overflow=Wrap  XmcBlockStatus=1  maskContainerNames=tabcontainer1  block_type=mux  block_config=sysgen:Mux_config
  Sum : hdlBasic/Logical  logical_function=OR  inputs=4  en=off  latency=0  precision=Full  arith_type=Unsigned  n_bits=16  bin_pt=0  align_bp=on  overflow=[]  quantization=[]  XmcBlockStatus=1  maskContainerNames=tabcontainer1  block_type=logical  block_config=sysgen:Logical_config
  c_out : hdlBasic/Logical  logical_function=OR  inputs=3  en=off  latency=0  precision=Full  arith_type=Unsigned  n_bits=16  bin_pt=0  align_bp=on  overflow=[]  quantization=[]  XmcBlockStatus=1  maskContainerNames=tabcontainer1  block_type=logical  block_config=sysgen:Logical_config
  ALU_OUT (1 BIT) : Outport
  CARRY_OUT (1 BIT) : Outport  Port=2
  SET (1 BIT) : Outport  Port=3
  wires:
  Mux1/1 -> Logical3/1, Logical7/1, Inverter8/1, Logical5/2, Logical/2, Logical2/1, Logical9/2
  Logical1/1 -> c_out/2
  Inverter8/1 -> Logical6/2, Logical4/2
  A_INPUT (1 BIT)/1 -> Mux1/2, Inverter2/1
  CARRY_IN (1 BIT)/1 -> Inverter1/1, Logical5/1, Logical4/1, Logical1/1, Logical/1
  Mux2/1 -> Logical5/3, Logical6/3, Logical1/2, Logical2/2, Inverter9/1, Logical3/2, Logical7/2
  Inverter2/1 -> Mux1/3
  Inverter1/1 -> Logical6/1, Logical9/1
  Logical6/1 -> Sum/3
  B_INPUT (1 BIT)/1 -> Inverter3/1, Mux2/2
  Logical9/1 -> Sum/2
  Sum/1 -> SET (1 BIT)/1, Mux/4
  Logical4/1 -> Sum/1
  Inverter3/1 -> Mux2/3
  Logical7/1 -> Mux/3
  Logical/1 -> c_out/1
  Logical5/1 -> Sum/4
  Logical3/1 -> Mux/2
  Inverter9/1 -> Logical9/3, Logical4/3
  Mux/1 -> ALU_OUT (1 BIT)/1
  Logical2/1 -> c_out/3
  OP (2 BIT)/1 -> Mux/1
  A_INVERT (1 BIT)/1 -> Mux1/1
  B_INVERT (1 BIT)/1 -> Mux2/1
  c_out/1 -> CARRY_OUT (1 BIT)/1
  LESS (1 BIT)/1 -> Mux/5

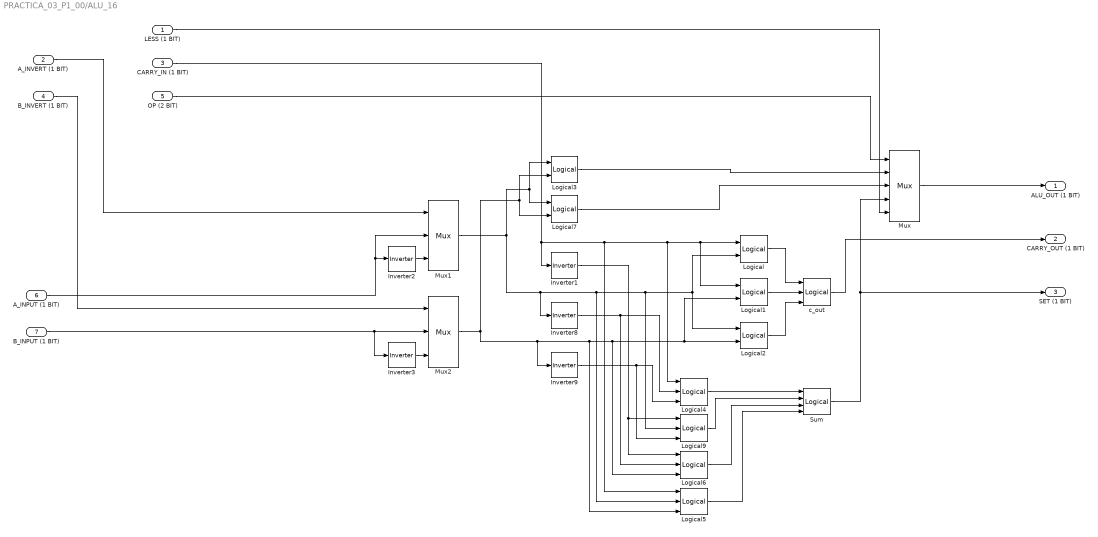
== system PRACTICA_03_P1_00/ALU_16 ==
  LESS (1 BIT) : Inport
  A_INVERT (1 BIT) : Inport  Port=2
  CARRY_IN (1 BIT) : Inport  Port=3
  B_INVERT (1 BIT) : Inport  Port=4
  OP (2 BIT) : Inport  Port=5
  A_INPUT (1 BIT) : Inport  Port=6
  B_INPUT (1 BIT) : Inport  Port=7
  Inverter{1..3,8..9} (5 alike) : hdlBasic/Inverter  en=off  latency=0  XmcBlockStatus=1  maskContainerNames=group2  block_type=inv  block_config=sysgen:Inverter_config
  Logical{,1..3} (4 alike) : hdlBasic/Logical  logical_function=AND  inputs=2  en=off  latency=0  precision=Full  arith_type=Unsigned  n_bits=16  bin_pt=0  align_bp=on  overflow=[]  quantization=[]  XmcBlockStatus=1  maskContainerNames=tabcontainer1  block_type=logical  block_config=sysgen:Logical_config
  Logical{4..6,9} (4 alike) : hdlBasic/Logical  logical_function=AND  inputs=3  en=off  latency=0  precision=Full  arith_type=Unsigned  n_bits=16  bin_pt=0  align_bp=on  overflow=[]  quantization=[]  XmcBlockStatus=1  maskContainerNames=tabcontainer1  block_type=logical  block_config=sysgen:Logical_config
  Logical7 : hdlBasic/Logical  logical_function=OR  inputs=2  en=off  latency=0  precision=Full  arith_type=Unsigned  n_bits=16  bin_pt=0  align_bp=on  overflow=[]  quantization=[]  XmcBlockStatus=1  maskContainerNames=tabcontainer1  block_type=logical  block_config=sysgen:Logical_config
  Mux : hdlBasic/Mux  inputs=4  en=off  latency=0  precision=Full  arith_type=Unsigned  n_bits=16  bin_pt=14  quantization=Truncate  overflow=Wrap  XmcBlockStatus=1  maskContainerNames=tabcontainer1  block_type=mux  block_config=sysgen:Mux_config
  Mux1 : hdlBasic/Mux  inputs=2  en=off  latency=0  precision=Full  arith_type=Unsigned  n_bits=16  bin_pt=14  quantization=Truncate  overflow=Wrap  XmcBlockStatus=1  maskContainerNames=tabcontainer1  block_type=mux  block_config=sysgen:Mux_config
  Mux2 : hdlBasic/Mux  inputs=2  en=off  latency=0  precision=Full  arith_type=Unsigned  n_bits=16  bin_pt=14  quantization=Truncate  overflow=Wrap  XmcBlockStatus=1  maskContainerNames=tabcontainer1  block_type=mux  block_config=sysgen:Mux_config
  Sum : hdlBasic/Logical  logical_function=OR  inputs=4  en=off  latency=0  precision=Full  arith_type=Unsigned  n_bits=16  bin_pt=0  align_bp=on  overflow=[]  quantization=[]  XmcBlockStatus=1  maskContainerNames=tabcontainer1  block_type=logical  block_config=sysgen:Logical_config
  c_out : hdlBasic/Logical  logical_function=OR  inputs=3  en=off  latency=0  precision=Full  arith_type=Unsigned  n_bits=16  bin_pt=0  align_bp=on  overflow=[]  quantization=[]  XmcBlockStatus=1  maskContainerNames=tabcontainer1  block_type=logical  block_config=sysgen:Logical_config
  ALU_OUT (1 BIT) : Outport
  CARRY_OUT (1 BIT) : Outport  Port=2
  SET (1 BIT) : Outport  Port=3
  wires:
  Mux1/1 -> Logical3/1, Logical7/1, Inverter8/1, Logical5/2, Logical/2, Logical2/1, Logical9/2
  Logical1/1 -> c_out/2
  Inverter8/1 -> Logical6/2, Logical4/2
  A_INPUT (1 BIT)/1 -> Mux1/2, Inverter2/1
  CARRY_IN (1 BIT)/1 -> Inverter1/1, Logical5/1, Logical4/1, Logical1/1, Logical/1
  Mux2/1 -> Logical5/3, Logical6/3, Logical1/2, Logical2/2, Inverter9/1, Logical3/2, Logical7/2
  Inverter2/1 -> Mux1/3
  Inverter1/1 -> Logical6/1, Logical9/1
  Logical6/1 -> Sum/3
  B_INPUT (1 BIT)/1 -> Inverter3/1, Mux2/2
  Logical9/1 -> Sum/2
  Sum/1 -> SET (1 BIT)/1, Mux/4
  Logical4/1 -> Sum/1
  Inverter3/1 -> Mux2/3
  Logical7/1 -> Mux/3
  Logical/1 -> c_out/1
  Logical5/1 -> Sum/4
  Logical3/1 -> Mux/2
  Inverter9/1 -> Logical9/3, Logical4/3
  Mux/1 -> ALU_OUT (1 BIT)/1
  Logical2/1 -> c_out/3
  OP (2 BIT)/1 -> Mux/1
  A_INVERT (1 BIT)/1 -> Mux1/1
  B_INVERT (1 BIT)/1 -> Mux2/1
  c_out/1 -> CARRY_OUT (1 BIT)/1
  LESS (1 BIT)/1 -> Mux/5

== system PRACTICA_03_P1_00/ALU_17 ==
  LESS (1 BIT) : Inport
  A_INVERT (1 BIT) : Inport  Port=2
  CARRY_IN (1 BIT) : Inport  Port=3
  B_INVERT (1 BIT) : Inport  Port=4
  OP (2 BIT) : Inport  Port=5
  A_INPUT (1 BIT) : Inport  Port=6
  B_INPUT (1 BIT) : Inport  Port=7
  Inverter{1..3,8..9} (5 alike) : hdlBasic/Inverter  en=off  latency=0  XmcBlockStatus=1  maskContainerNames=group2  block_type=inv  block_config=sysgen:Inverter_config
  Logical{,1..3} (4 alike) : hdlBasic/Logical  logical_function=AND  inputs=2  en=off  latency=0  precision=Full  arith_type=Unsigned  n_bits=16  bin_pt=0  align_bp=on  overflow=[]  quantization=[]  XmcBlockStatus=1  maskContainerNames=tabcontainer1  block_type=logical  block_config=sysgen:Logical_config
  Logical{4..6,9} (4 alike) : hdlBasic/Logical  logical_function=AND  inputs=3  en=off  latency=0  precision=Full  arith_type=Unsigned  n_bits=16  bin_pt=0  align_bp=on  overflow=[]  quantization=[]  XmcBlockStatus=1  maskContainerNames=tabcontainer1  block_type=logical  block_config=sysgen:Logical_config
  Logical7 : hdlBasic/Logical  logical_function=OR  inputs=2  en=off  latency=0  precision=Full  arith_type=Unsigned  n_bits=16  bin_pt=0  align_bp=on  overflow=[]  quantization=[]  XmcBlockStatus=1  maskContainerNames=tabcontainer1  block_type=logical  block_config=sysgen:Logical_config
  Mux : hdlBasic/Mux  inputs=4  en=off  latency=0  precision=Full  arith_type=Unsigned  n_bits=16  bin_pt=14  quantization=Truncate  overflow=Wrap  XmcBlockStatus=1  maskContainerNames=tabcontainer1  block_type=mux  block_config=sysgen:Mux_config
  Mux1 : hdlBasic/Mux  inputs=2  en=off  latency=0  precision=Full  arith_type=Unsigned  n_bits=16  bin_pt=14  quantization=Truncate  overflow=Wrap  XmcBlockStatus=1  maskContainerNames=tabcontainer1  block_type=mux  block_config=sysgen:Mux_config
  Mux2 : hdlBasic/Mux  inputs=2  en=off  latency=0  precision=Full  arith_type=Unsigned  n_bits=16  bin_pt=14  quantization=Truncate  overflow=Wrap  XmcBlockStatus=1  maskContainerNames=tabcontainer1  block_type=mux  block_config=sysgen:Mux_config
  Sum : hdlBasic/Logical  logical_function=OR  inputs=4  en=off  latency=0  precision=Full  arith_type=Unsigned  n_bits=16  bin_pt=0  align_bp=on  overflow=[]  quantization=[]  XmcBlockStatus=1  maskContainerNames=tabcontainer1  block_type=logical  block_config=sysgen:Logical_config
  c_out : hdlBasic/Logical  logical_function=OR  inputs=3  en=off  latency=0  precision=Full  arith_type=Unsigned  n_bits=16  bin_pt=0  align_bp=on  overflow=[]  quantization=[]  XmcBlockStatus=1  maskContainerNames=tabcontainer1  block_type=logical  block_config=sysgen:Logical_config
  ALU_OUT (1 BIT) : Outport
  CARRY_OUT (1 BIT) : Outport  Port=2
  SET (1 BIT) : Outport  Port=3
  wires:
  Mux1/1 -> Logical3/1, Logical7/1, Inverter8/1, Logical5/2, Logical/2, Logical2/1, Logical9/2
  Logical1/1 -> c_out/2
  Inverter8/1 -> Logical6/2, Logical4/2
  A_INPUT (1 BIT)/1 -> Mux1/2, Inverter2/1
  CARRY_IN (1 BIT)/1 -> Inverter1/1, Logical5/1, Logical4/1, Logical1/1, Logical/1
  Mux2/1 -> Logical5/3, Logical6/3, Logical1/2, Logical2/2, Inverter9/1, Logical3/2, Logical7/2
  Inverter2/1 -> Mux1/3
  Inverter1/1 -> Logical6/1, Logical9/1
  Logical6/1 -> Sum/3
  B_INPUT (1 BIT)/1 -> Inverter3/1, Mux2/2
  Logical9/1 -> Sum/2
  Sum/1 -> SET (1 BIT)/1, Mux/4
  Logical4/1 -> Sum/1
  Inverter3/1 -> Mux2/3
  Logical7/1 -> Mux/3
  Logical/1 -> c_out/1
  Logical5/1 -> Sum/4
  Logical3/1 -> Mux/2
  Inverter9/1 -> Logical9/3, Logical4/3
  Mux/1 -> ALU_OUT (1 BIT)/1
  Logical2/1 -> c_out/3
  OP (2 BIT)/1 -> Mux/1
  A_INVERT (1 BIT)/1 -> Mux1/1
  B_INVERT (1 BIT)/1 -> Mux2/1
  c_out/1 -> CARRY_OUT (1 BIT)/1
  LESS (1 BIT)/1 -> Mux/5

== system PRACTICA_03_P1_00/ALU_18 ==
  LESS (1 BIT) : Inport
  A_INVERT (1 BIT) : Inport  Port=2
  CARRY_IN (1 BIT) : Inport  Port=3
  B_INVERT (1 BIT) : Inport  Port=4
  OP (2 BIT) : Inport  Port=5
  A_INPUT (1 BIT) : Inport  Port=6
  B_INPUT (1 BIT) : Inport  Port=7
  Inverter{1..3,8..9} (5 alike) : hdlBasic/Inverter  en=off  latency=0  XmcBlockStatus=1  maskContainerNames=group2  block_type=inv  block_config=sysgen:Inverter_config
  Logical{,1..3} (4 alike) : hdlBasic/Logical  logical_function=AND  inputs=2  en=off  latency=0  precision=Full  arith_type=Unsigned  n_bits=16  bin_pt=0  align_bp=on  overflow=[]  quantization=[]  XmcBlockStatus=1  maskContainerNames=tabcontainer1  block_type=logical  block_config=sysgen:Logical_config
  Logical{4..6,9} (4 alike) : hdlBasic/Logical  logical_function=AND  inputs=3  en=off  latency=0  precision=Full  arith_type=Unsigned  n_bits=16  bin_pt=0  align_bp=on  overflow=[]  quantization=[]  XmcBlockStatus=1  maskContainerNames=tabcontainer1  block_type=logical  block_config=sysgen:Logical_config
  Logical7 : hdlBasic/Logical  logical_function=OR  inputs=2  en=off  latency=0  precision=Full  arith_type=Unsigned  n_bits=16  bin_pt=0  align_bp=on  overflow=[]  quantization=[]  XmcBlockStatus=1  maskContainerNames=tabcontainer1  block_type=logical  block_config=sysgen:Logical_config
  Mux : hdlBasic/Mux  inputs=4  en=off  latency=0  precision=Full  arith_type=Unsigned  n_bits=16  bin_pt=14  quantization=Truncate  overflow=Wrap  XmcBlockStatus=1  maskContainerNames=tabcontainer1  block_type=mux  block_config=sysgen:Mux_config
  Mux1 : hdlBasic/Mux  inputs=2  en=off  latency=0  precision=Full  arith_type=Unsigned  n_bits=16  bin_pt=14  quantization=Truncate  overflow=Wrap  XmcBlockStatus=1  maskContainerNames=tabcontainer1  block_type=mux  block_config=sysgen:Mux_config
  Mux2 : hdlBasic/Mux  inputs=2  en=off  latency=0  precision=Full  arith_type=Unsigned  n_bits=16  bin_pt=14  quantization=Truncate  overflow=Wrap  XmcBlockStatus=1  maskContainerNames=tabcontainer1  block_type=mux  block_config=sysgen:Mux_config
  Sum : hdlBasic/Logical  logical_function=OR  inputs=4  en=off  latency=0  precision=Full  arith_type=Unsigned  n_bits=16  bin_pt=0  align_bp=on  overflow=[]  quantization=[]  XmcBlockStatus=1  maskContainerNames=tabcontainer1  block_type=logical  block_config=sysgen:Logical_config
  c_out : hdlBasic/Logical  logical_function=OR  inputs=3  en=off  latency=0  precision=Full  arith_type=Unsigned  n_bits=16  bin_pt=0  align_bp=on  overflow=[]  quantization=[]  XmcBlockStatus=1  maskContainerNames=tabcontainer1  block_type=logical  block_config=sysgen:Logical_config
  ALU_OUT (1 BIT) : Outport
  CARRY_OUT (1 BIT) : Outport  Port=2
  SET (1 BIT) : Outport  Port=3
  wires:
  Mux1/1 -> Logical3/1, Logical7/1, Inverter8/1, Logical5/2, Logical/2, Logical2/1, Logical9/2
  Logical1/1 -> c_out/2
  Inverter8/1 -> Logical6/2, Logical4/2
  A_INPUT (1 BIT)/1 -> Mux1/2, Inverter2/1
  CARRY_IN (1 BIT)/1 -> Inverter1/1, Logical5/1, Logical4/1, Logical1/1, Logical/1
  Mux2/1 -> Logical5/3, Logical6/3, Logical1/2, Logical2/2, Inverter9/1, Logical3/2, Logical7/2
  Inverter2/1 -> Mux1/3
  Inverter1/1 -> Logical6/1, Logical9/1
  Logical6/1 -> Sum/3
  B_INPUT (1 BIT)/1 -> Inverter3/1, Mux2/2
  Logical9/1 -> Sum/2
  Sum/1 -> SET (1 BIT)/1, Mux/4
  Logical4/1 -> Sum/1
  Inverter3/1 -> Mux2/3
  Logical7/1 -> Mux/3
  Logical/1 -> c_out/1
  Logical5/1 -> Sum/4
  Logical3/1 -> Mux/2
  Inverter9/1 -> Logical9/3, Logical4/3
  Mux/1 -> ALU_OUT (1 BIT)/1
  Logical2/1 -> c_out/3
  OP (2 BIT)/1 -> Mux/1
  A_INVERT (1 BIT)/1 -> Mux1/1
  B_INVERT (1 BIT)/1 -> Mux2/1
  c_out/1 -> CARRY_OUT (1 BIT)/1
  LESS (1 BIT)/1 -> Mux/5

== system PRACTICA_03_P1_00/ALU_19 ==
  LESS (1 BIT) : Inport
  A_INVERT (1 BIT) : Inport  Port=2
  CARRY_IN (1 BIT) : Inport  Port=3
  B_INVERT (1 BIT) : Inport  Port=4
  OP (2 BIT) : Inport  Port=5
  A_INPUT (1 BIT) : Inport  Port=6
  B_INPUT (1 BIT) : Inport  Port=7
  Inverter{1..3,8..9} (5 alike) : hdlBasic/Inverter  en=off  latency=0  XmcBlockStatus=1  maskContainerNames=group2  block_type=inv  block_config=sysgen:Inverter_config
  Logical{,1..3} (4 alike) : hdlBasic/Logical  logical_function=AND  inputs=2  en=off  latency=0  precision=Full  arith_type=Unsigned  n_bits=16  bin_pt=0  align_bp=on  overflow=[]  quantization=[]  XmcBlockStatus=1  maskContainerNames=tabcontainer1  block_type=logical  block_config=sysgen:Logical_config
  Logical{4..6,9} (4 alike) : hdlBasic/Logical  logical_function=AND  inputs=3  en=off  latency=0  precision=Full  arith_type=Unsigned  n_bits=16  bin_pt=0  align_bp=on  overflow=[]  quantization=[]  XmcBlockStatus=1  maskContainerNames=tabcontainer1  block_type=logical  block_config=sysgen:Logical_config
  Logical7 : hdlBasic/Logical  logical_function=OR  inputs=2  en=off  latency=0  precision=Full  arith_type=Unsigned  n_bits=16  bin_pt=0  align_bp=on  overflow=[]  quantization=[]  XmcBlockStatus=1  maskContainerNames=tabcontainer1  block_type=logical  block_config=sysgen:Logical_config
  Mux : hdlBasic/Mux  inputs=4  en=off  latency=0  precision=Full  arith_type=Unsigned  n_bits=16  bin_pt=14  quantization=Truncate  overflow=Wrap  XmcBlockStatus=1  maskContainerNames=tabcontainer1  block_type=mux  block_config=sysgen:Mux_config
  Mux1 : hdlBasic/Mux  inputs=2  en=off  latency=0  precision=Full  arith_type=Unsigned  n_bits=16  bin_pt=14  quantization=Truncate  overflow=Wrap  XmcBlockStatus=1  maskContainerNames=tabcontainer1  block_type=mux  block_config=sysgen:Mux_config
  Mux2 : hdlBasic/Mux  inputs=2  en=off  latency=0  precision=Full  arith_type=Unsigned  n_bits=16  bin_pt=14  quantization=Truncate  overflow=Wrap  XmcBlockStatus=1  maskContainerNames=tabcontainer1  block_type=mux  block_config=sysgen:Mux_config
  Sum : hdlBasic/Logical  logical_function=OR  inputs=4  en=off  latency=0  precision=Full  arith_type=Unsigned  n_bits=16  bin_pt=0  align_bp=on  overflow=[]  quantization=[]  XmcBlockStatus=1  maskContainerNames=tabcontainer1  block_type=logical  block_config=sysgen:Logical_config
  c_out : hdlBasic/Logical  logical_function=OR  inputs=3  en=off  latency=0  precision=Full  arith_type=Unsigned  n_bits=16  bin_pt=0  align_bp=on  overflow=[]  quantization=[]  XmcBlockStatus=1  maskContainerNames=tabcontainer1  block_type=logical  block_config=sysgen:Logical_config
  ALU_OUT (1 BIT) : Outport
  CARRY_OUT (1 BIT) : Outport  Port=2
  SET (1 BIT) : Outport  Port=3
  wires:
  Mux1/1 -> Logical3/1, Logical7/1, Inverter8/1, Logical5/2, Logical/2, Logical2/1, Logical9/2
  Logical1/1 -> c_out/2
  Inverter8/1 -> Logical6/2, Logical4/2
  A_INPUT (1 BIT)/1 -> Mux1/2, Inverter2/1
  CARRY_IN (1 BIT)/1 -> Inverter1/1, Logical5/1, Logical4/1, Logical1/1, Logical/1
  Mux2/1 -> Logical5/3, Logical6/3, Logical1/2, Logical2/2, Inverter9/1, Logical3/2, Logical7/2
  Inverter2/1 -> Mux1/3
  Inverter1/1 -> Logical6/1, Logical9/1
  Logical6/1 -> Sum/3
  B_INPUT (1 BIT)/1 -> Inverter3/1, Mux2/2
  Logical9/1 -> Sum/2
  Sum/1 -> SET (1 BIT)/1, Mux/4
  Logical4/1 -> Sum/1
  Inverter3/1 -> Mux2/3
  Logical7/1 -> Mux/3
  Logical/1 -> c_out/1
  Logical5/1 -> Sum/4
  Logical3/1 -> Mux/2
  Inverter9/1 -> Logical9/3, Logical4/3
  Mux/1 -> ALU_OUT (1 BIT)/1
  Logical2/1 -> c_out/3
  OP (2 BIT)/1 -> Mux/1
  A_INVERT (1 BIT)/1 -> Mux1/1
  B_INVERT (1 BIT)/1 -> Mux2/1
  c_out/1 -> CARRY_OUT (1 BIT)/1
  LESS (1 BIT)/1 -> Mux/5

== system PRACTICA_03_P1_00/ALU_2 ==
  LESS (1 BIT) : Inport
  A_INVERT (1 BIT) : Inport  Port=2
  CARRY_IN (1 BIT) : Inport  Port=3
  B_INVERT (1 BIT) : Inport  Port=4
  OP (2 BIT) : Inport  Port=5
  A_INPUT (1 BIT) : Inport  Port=6
  B_INPUT (1 BIT) : Inport  Port=7
  Inverter{1..3,8..9} (5 alike) : hdlBasic/Inverter  en=off  latency=0  XmcBlockStatus=1  maskContainerNames=group2  block_type=inv  block_config=sysgen:Inverter_config
  Logical{,1..3} (4 alike) : hdlBasic/Logical  logical_function=AND  inputs=2  en=off  latency=0  precision=Full  arith_type=Unsigned  n_bits=16  bin_pt=0  align_bp=on  overflow=[]  quantization=[]  XmcBlockStatus=1  maskContainerNames=tabcontainer1  block_type=logical  block_config=sysgen:Logical_config
  Logical{4..6,9} (4 alike) : hdlBasic/Logical  logical_function=AND  inputs=3  en=off  latency=0  precision=Full  arith_type=Unsigned  n_bits=16  bin_pt=0  align_bp=on  overflow=[]  quantization=[]  XmcBlockStatus=1  maskContainerNames=tabcontainer1  block_type=logical  block_config=sysgen:Logical_config
  Logical7 : hdlBasic/Logical  logical_function=OR  inputs=2  en=off  latency=0  precision=Full  arith_type=Unsigned  n_bits=16  bin_pt=0  align_bp=on  overflow=[]  quantization=[]  XmcBlockStatus=1  maskContainerNames=tabcontainer1  block_type=logical  block_config=sysgen:Logical_config
  Mux : hdlBasic/Mux  inputs=4  en=off  latency=0  precision=Full  arith_type=Unsigned  n_bits=16  bin_pt=14  quantization=Truncate  overflow=Wrap  XmcBlockStatus=1  maskContainerNames=tabcontainer1  block_type=mux  block_config=sysgen:Mux_config
  Mux1 : hdlBasic/Mux  inputs=2  en=off  latency=0  precision=Full  arith_type=Unsigned  n_bits=16  bin_pt=14  quantization=Truncate  overflow=Wrap  XmcBlockStatus=1  maskContainerNames=tabcontainer1  block_type=mux  block_config=sysgen:Mux_config
  Mux2 : hdlBasic/Mux  inputs=2  en=off  latency=0  precision=Full  arith_type=Unsigned  n_bits=16  bin_pt=14  quantization=Truncate  overflow=Wrap  XmcBlockStatus=1  maskContainerNames=tabcontainer1  block_type=mux  block_config=sysgen:Mux_config
  Sum : hdlBasic/Logical  logical_function=OR  inputs=4  en=off  latency=0  precision=Full  arith_type=Unsigned  n_bits=16  bin_pt=0  align_bp=on  overflow=[]  quantization=[]  XmcBlockStatus=1  maskContainerNames=tabcontainer1  block_type=logical  block_config=sysgen:Logical_config
  c_out : hdlBasic/Logical  logical_function=OR  inputs=3  en=off  latency=0  precision=Full  arith_type=Unsigned  n_bits=16  bin_pt=0  align_bp=on  overflow=[]  quantization=[]  XmcBlockStatus=1  maskContainerNames=tabcontainer1  block_type=logical  block_config=sysgen:Logical_config
  ALU_OUT (1 BIT) : Outport
  CARRY_OUT (1 BIT) : Outport  Port=2
  SET (1 BIT) : Outport  Port=3
  wires:
  Mux1/1 -> Logical3/1, Logical7/1, Inverter8/1, Logical5/2, Logical/2, Logical2/1, Logical9/2
  Logical1/1 -> c_out/2
  Inverter8/1 -> Logical6/2, Logical4/2
  A_INPUT (1 BIT)/1 -> Mux1/2, Inverter2/1
  CARRY_IN (1 BIT)/1 -> Inverter1/1, Logical5/1, Logical4/1, Logical1/1, Logical/1
  Mux2/1 -> Logical5/3, Logical6/3, Logical1/2, Logical2/2, Inverter9/1, Logical3/2, Logical7/2
  Inverter2/1 -> Mux1/3
  Inverter1/1 -> Logical6/1, Logical9/1
  Logical6/1 -> Sum/3
  B_INPUT (1 BIT)/1 -> Inverter3/1, Mux2/2
  Logical9/1 -> Sum/2
  Sum/1 -> SET (1 BIT)/1, Mux/4
  Logical4/1 -> Sum/1
  Inverter3/1 -> Mux2/3
  Logical7/1 -> Mux/3
  Logical/1 -> c_out/1
  Logical5/1 -> Sum/4
  Logical3/1 -> Mux/2
  Inverter9/1 -> Logical9/3, Logical4/3
  Mux/1 -> ALU_OUT (1 BIT)/1
  Logical2/1 -> c_out/3
  OP (2 BIT)/1 -> Mux/1
  A_INVERT (1 BIT)/1 -> Mux1/1
  B_INVERT (1 BIT)/1 -> Mux2/1
  c_out/1 -> CARRY_OUT (1 BIT)/1
  LESS (1 BIT)/1 -> Mux/5

== system PRACTICA_03_P1_00/ALU_20 ==
  LESS (1 BIT) : Inport
  A_INVERT (1 BIT) : Inport  Port=2
  CARRY_IN (1 BIT) : Inport  Port=3
  B_INVERT (1 BIT) : Inport  Port=4
  OP (2 BIT) : Inport  Port=5
  A_INPUT (1 BIT) : Inport  Port=6
  B_INPUT (1 BIT) : Inport  Port=7
  Inverter{1..3,8..9} (5 alike) : hdlBasic/Inverter  en=off  latency=0  XmcBlockStatus=1  maskContainerNames=group2  block_type=inv  block_config=sysgen:Inverter_config
  Logical{,1..3} (4 alike) : hdlBasic/Logical  logical_function=AND  inputs=2  en=off  latency=0  precision=Full  arith_type=Unsigned  n_bits=16  bin_pt=0  align_bp=on  overflow=[]  quantization=[]  XmcBlockStatus=1  maskContainerNames=tabcontainer1  block_type=logical  block_config=sysgen:Logical_config
  Logical{4..6,9} (4 alike) : hdlBasic/Logical  logical_function=AND  inputs=3  en=off  latency=0  precision=Full  arith_type=Unsigned  n_bits=16  bin_pt=0  align_bp=on  overflow=[]  quantization=[]  XmcBlockStatus=1  maskContainerNames=tabcontainer1  block_type=logical  block_config=sysgen:Logical_config
  Logical7 : hdlBasic/Logical  logical_function=OR  inputs=2  en=off  latency=0  precision=Full  arith_type=Unsigned  n_bits=16  bin_pt=0  align_bp=on  overflow=[]  quantization=[]  XmcBlockStatus=1  maskContainerNames=tabcontainer1  block_type=logical  block_config=sysgen:Logical_config
  Mux : hdlBasic/Mux  inputs=4  en=off  latency=0  precision=Full  arith_type=Unsigned  n_bits=16  bin_pt=14  quantization=Truncate  overflow=Wrap  XmcBlockStatus=1  maskContainerNames=tabcontainer1  block_type=mux  block_config=sysgen:Mux_config
  Mux1 : hdlBasic/Mux  inputs=2  en=off  latency=0  precision=Full  arith_type=Unsigned  n_bits=16  bin_pt=14  quantization=Truncate  overflow=Wrap  XmcBlockStatus=1  maskContainerNames=tabcontainer1  block_type=mux  block_config=sysgen:Mux_config
  Mux2 : hdlBasic/Mux  inputs=2  en=off  latency=0  precision=Full  arith_type=Unsigned  n_bits=16  bin_pt=14  quantization=Truncate  overflow=Wrap  XmcBlockStatus=1  maskContainerNames=tabcontainer1  block_type=mux  block_config=sysgen:Mux_config
  Sum : hdlBasic/Logical  logical_function=OR  inputs=4  en=off  latency=0  precision=Full  arith_type=Unsigned  n_bits=16  bin_pt=0  align_bp=on  overflow=[]  quantization=[]  XmcBlockStatus=1  maskContainerNames=tabcontainer1  block_type=logical  block_config=sysgen:Logical_config
  c_out : hdlBasic/Logical  logical_function=OR  inputs=3  en=off  latency=0  precision=Full  arith_type=Unsigned  n_bits=16  bin_pt=0  align_bp=on  overflow=[]  quantization=[]  XmcBlockStatus=1  maskContainerNames=tabcontainer1  block_type=logical  block_config=sysgen:Logical_config
  ALU_OUT (1 BIT) : Outport
  CARRY_OUT (1 BIT) : Outport  Port=2
  SET (1 BIT) : Outport  Port=3
  wires:
  Mux1/1 -> Logical3/1, Logical7/1, Inverter8/1, Logical5/2, Logical/2, Logical2/1, Logical9/2
  Logical1/1 -> c_out/2
  Inverter8/1 -> Logical6/2, Logical4/2
  A_INPUT (1 BIT)/1 -> Mux1/2, Inverter2/1
  CARRY_IN (1 BIT)/1 -> Inverter1/1, Logical5/1, Logical4/1, Logical1/1, Logical/1
  Mux2/1 -> Logical5/3, Logical6/3, Logical1/2, Logical2/2, Inverter9/1, Logical3/2, Logical7/2
  Inverter2/1 -> Mux1/3
  Inverter1/1 -> Logical6/1, Logical9/1
  Logical6/1 -> Sum/3
  B_INPUT (1 BIT)/1 -> Inverter3/1, Mux2/2
  Logical9/1 -> Sum/2
  Sum/1 -> SET (1 BIT)/1, Mux/4
  Logical4/1 -> Sum/1
  Inverter3/1 -> Mux2/3
  Logical7/1 -> Mux/3
  Logical/1 -> c_out/1
  Logical5/1 -> Sum/4
  Logical3/1 -> Mux/2
  Inverter9/1 -> Logical9/3, Logical4/3
  Mux/1 -> ALU_OUT (1 BIT)/1
  Logical2/1 -> c_out/3
  OP (2 BIT)/1 -> Mux/1
  A_INVERT (1 BIT)/1 -> Mux1/1
  B_INVERT (1 BIT)/1 -> Mux2/1
  c_out/1 -> CARRY_OUT (1 BIT)/1
  LESS (1 BIT)/1 -> Mux/5
